simulink model "B5G_SIM_PDR_ASH_V0"  (R2021a)
settings: Solver=ode4  StartTime=0.0  StopTime=dm.duration  FixedStep=dm.dt  RelTol=1e-3
InitFcn:
  | %b5g_init_param_sdr_v1;
StopFcn:
  | %b5g_post_param_sdr_v1;
  | 
  | %if mdl.OpenAfterSim.sdi
  | %   Simulink.sdi.view;
  | %end
  | 
  | %if mdl.OpenAfterSim.Scope
  | %   open_system(strcat(gcs,'/RateRwTorque'));
  | %end
model workspace (MAT data in the model file):
  RWModelType = 0
values from neighbouring files (symbols this model uses):
  dm = set_dm(dm)    [INIT_B5G_SIM_PDR_ASH.m]
  mdl = set_model_control()    [INIT_B5G_SIM_PDR_ASH.m]    (also in init_b5g_sim_pdr.m = set_model_control('B5G_SIM_PDR_V1'))
  rads2rpm = 60/(2*pi)    (= 9.54929658551)    [INIT_B5G_SIM_PDR_ASH.m]    (also in init_b5g_sim_pdr.m)
undefined symbols (not defined in the file or in its folder): Eclipse, fsw, MagSc, PVeci, Qi2b, RateSc, SunSc
libraries: vrlib x2, aerolibtransform2 x1
(part 1 of 2)
settings Model: SimulationMode=accelerator  ParameterArgumentNames=RWModelType  OrderedModelArguments=off  Creator=Jack-AOCS  LastModifiedBy=jacky
settings SolverCC: AlgebraicLoopSolver=TrustRegion  MinimalZcImpactIntegration=on
settings DataIOCC: SaveFormat=Array
settings OptimizationCC: AccelVerboseBuild=on
settings DebuggingCC: ReadBeforeWriteMsg=DisableAll  WriteAfterWriteMsg=DisableAll  WriteAfterReadMsg=DisableAll  MultiTaskDSMMsg=none  SFMachineParentedDataDiag=warning  ArithmeticOperatorsInVariantConditions=warning
settings ModelReferenceCC: UpdateModelReferenceTargets=IfOutOfDate
settings SFSimCC: SFSimEcho=off  SimUseLocalCustomCode=off  CustomCodeUndefinedFunction=UseInterfaceOnly
settings RTWCC: RTWUseLocalCustomCode=off

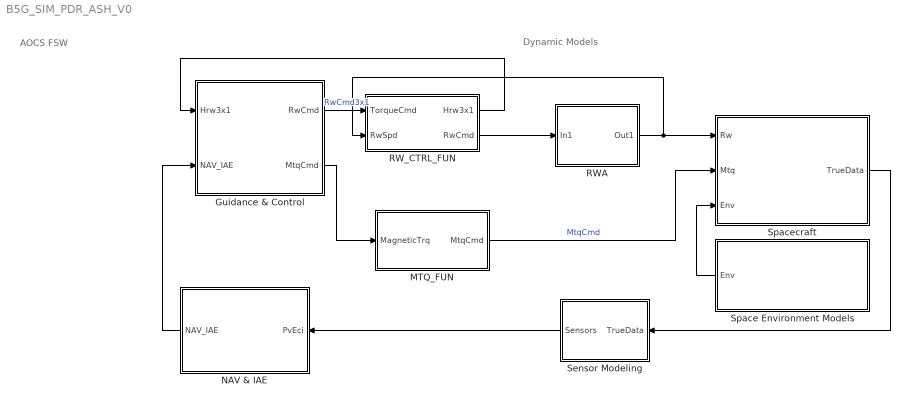
== system B5G_SIM_PDR_ASH_V0 ==
  note: AOCS FSW
  note: Dynamic Models
  Guidance & Control : Subsystem
  MTQ_FUN : Subsystem
  NAV & IAE : Subsystem
  RWA : Subsystem  Variant=on
  RW_CTRL_FUN : Subsystem
  Sensor Modeling : Subsystem
  Space Environment Models : Subsystem
  Spacecraft : Subsystem
  wires:
  Sensor Modeling/1(Sensors) -> NAV & IAE/1(PvEci)
  RWA/1(Out1) -> Spacecraft/1(Rw), RW_CTRL_FUN/2(RwSpd)
  Space Environment Models/1(Env) -> Spacecraft/3(Env)
  Spacecraft/1(TrueData) -> Sensor Modeling/1("TrueData ")
  RW_CTRL_FUN/2(RwCmd) -> RWA/1(In1)
  RW_CTRL_FUN/1(Hrw3x1) -> Guidance & Control/1(Hrw3x1)
  NAV & IAE/1(NAV_IAE) -> Guidance & Control/2(NAV_IAE)
  Guidance & Control/1(RwCmd) -> RW_CTRL_FUN/1(TorqueCmd)  "RwCmd3x1"
  Guidance & Control/2(MtqCmd) -> MTQ_FUN/1(MagneticTrq)
  MTQ_FUN/1(MtqCmd) -> Spacecraft/2(Mtq)  "MtqCmd"

== system B5G_SIM_PDR_ASH_V0/Guidance & Control ==
  Hrw3x1 : Inport
  NAV_IAE : Inport  Port=2
  ASH Mode : Subsystem
  RwCmd : Outport
  MtqCmd : Outport  Port=2
  wires:
  Hrw3x1/1 -> ASH Mode/1(Hrw3x1)
  NAV_IAE/1 -> ASH Mode/2(Sensors)
  ASH Mode/1(RwCmd) -> RwCmd/1  "RwTrq3"
  ASH Mode/2(MtqCmd) -> MtqCmd/1

== system B5G_SIM_PDR_ASH_V0/MTQ_FUN ==
  MagneticTrq : Inport
  Rate Transition : RateTransition  OutPortSampleTime=fsw.bdot_period
  Saturation : Saturate  UpperLimit=fsw.mtq.func.max_dipole  LowerLimit=-fsw.mtq.func.max_dipole
  MtqCmd : Outport
  wires:
  Rate Transition/1 -> Saturation/1
  Saturation/1 -> MtqCmd/1
  MagneticTrq/1 -> Rate Transition/1

== system B5G_SIM_PDR_ASH_V0/NAV & IAE ==
  PvEci : Inport
  Bus Creator : BusCreator  Inputs=2
  Bus Selector1 : BusSelector  OutputSignals=PVeci
  MATLAB Function : MATLAB Function  TreatAsAtomicUnit=on
  NAV_IAE : Outport
  wires:
  Bus Selector1/1 -> MATLAB Function/1(pv_eci)  "<PVeci>"
  PvEci/1 -> Bus Creator/2, Bus Selector1/1
  MATLAB Function/1(nav_out) -> Bus Creator/1
  Bus Creator/1 -> NAV_IAE/1

== system B5G_SIM_PDR_ASH_V0/RWA ==
  note: 1) Add Subsystem or Model blocks as valid variant choices.
      | 2) You cannot connect blocks at this level. At simulation, connectivity is automatically
      | determined, based on the active variant and port name matching.
  In1 : Inport
  Nonlinear : Subsystem  VariantControl=RWModel == 2
  Original : Subsystem  VariantControl=RWModel == 1
  Out1 : Outport

== system B5G_SIM_PDR_ASH_V0/RW_CTRL_FUN ==
  TorqueCmd : Inport
  RwSpd : Inport  Port=2
  Angular momentum Estimate : MATLAB Function  TreatAsAtomicUnit=on
  ComputeSaturate : MATLAB Function  TreatAsAtomicUnit=on
  D : Gain  Gain=fsw.rw.func.D  Multiplication=Matrix(K*u) (u vector)
  G : Gain  Gain=fsw.rw.func.G  Multiplication=Matrix(K*u) (u vector)
  RW Kernel Control : Subsystem
  Rate Transition : RateTransition  OutPortSampleTime=fsw.dt
  Sum2 : Sum  Inputs=|++
  Unit Delay : UnitDelay  SampleTime=-1  HasFrameUpgradeWarning=on
  Hrw3x1 : Outport
  RwCmd : Outport  Port=2
  wires:
  TorqueCmd/1 -> G/1
  RwSpd/1 -> Angular momentum Estimate/1(w_rpm)  "RwSpd"
  G/1 -> Sum2/1  "C_A"
  Sum2/1 -> ComputeSaturate/1(T)
  Angular momentum Estimate/1(h) -> D/1, RW Kernel Control/1(h_est)  "h_est"
  Unit Delay/1 -> Angular momentum Estimate/2(tc)
  RW Kernel Control/1(C_N) -> Sum2/2
  ComputeSaturate/1(Tc) -> Rate Transition/1, Unit Delay/1
  Rate Transition/1 -> RwCmd/1  "RwTrq4"
  D/1 -> Hrw3x1/1  "Hrw"

== system B5G_SIM_PDR_ASH_V0/Sensor Modeling ==
  "TrueData " : Inport
  Bus Creator : BusCreator  Inputs=5
  Bus Selector : BusSelector  OutputSignals=SunSc,Eclipse
  Bus Selector1 : BusSelector  OutputSignals=RateSc,Qi2b,MagSc,PVeci
  MATLAB Function : MATLAB Function  TreatAsAtomicUnit=on
  Sensors : Outport
  wires:
  "TrueData "/1 -> Bus Selector1/1, Bus Selector/1
  Bus Selector/1 -> MATLAB Function/1(SunSc)  "<SunSc>"
  Bus Selector/2 -> MATLAB Function/2(EclipFlag)  "<Eclipse>"
  MATLAB Function/1(SS_TM) -> Bus Creator/1
  Bus Selector1/1 -> Bus Creator/2  "<RateSc>"
  Bus Selector1/2 -> Bus Creator/3  "<Qi2b>"
  Bus Selector1/3 -> Bus Creator/4  "<MagSc>"
  Bus Selector1/4 -> Bus Creator/5  "<PVeci>"
  Bus Creator/1 -> Sensors/1

== system B5G_SIM_PDR_ASH_V0/Space Environment Models ==
  Bus Creator : BusCreator  Inputs=4
  ECI2ECF : MATLAB Function  TreatAsAtomicUnit=on
  Eclipse Condition : MATLAB Function  TreatAsAtomicUnit=on
  MagneticField : Subsystem
  Mux : Mux  Inputs=2
  "Orbit Propagator " : Subsystem
  Product : Product  Multiplication=Matrix(*)
  Sun Model : MATLAB Function  TreatAsAtomicUnit=on
  Timer : Subsystem
  Env : Outport  VectorParamsAs1DForOutWhenUnconnected=off
  wires:
  ECI2ECF/1(Rf2i) -> Product/1
  Product/1 -> Bus Creator/1  "Beci"
  "Orbit Propagator "/1(Peci) -> ECI2ECF/2(Peci), Mux/1
  "Orbit Propagator "/2(Veci) -> Mux/2
  Timer/1(JD) -> Sun Model/1(jD), ECI2ECF/1(jdut1)
  Mux/1 -> Eclipse Condition/2(PvEci), Bus Creator/4  "PVeci"
  Bus Creator/1 -> Env/1
  Sun Model/1(SunEci) -> Bus Creator/2, Eclipse Condition/1(SunEci)  "SunVeci"
  Eclipse Condition/1(EclipFlag) -> Bus Creator/3  "Eclipse"
  ECI2ECF/2(Pecf) -> MagneticField/1(In1)
  MagneticField/1(Out1) -> Product/2

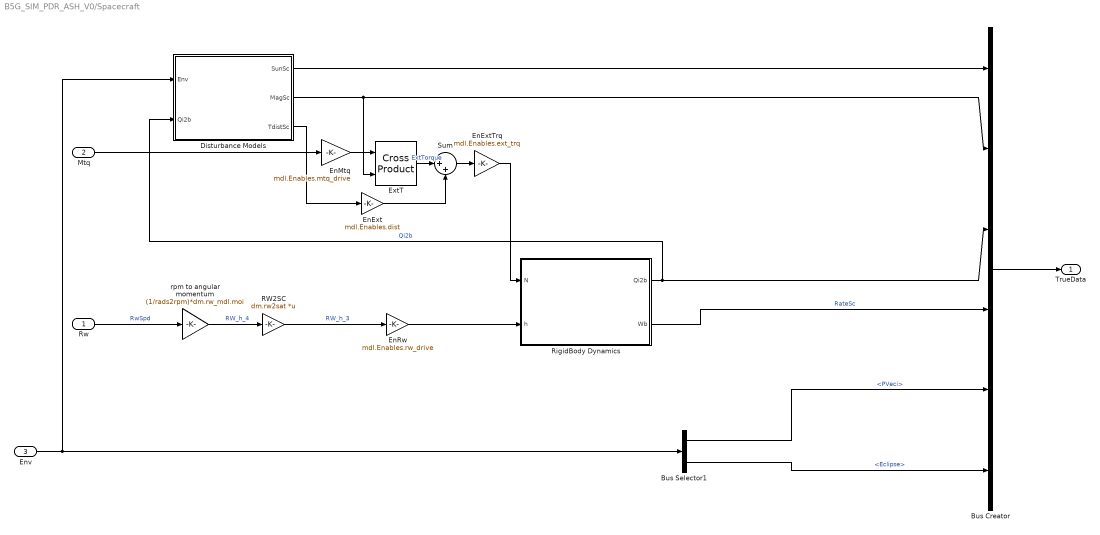
== system B5G_SIM_PDR_ASH_V0/Spacecraft ==
  Rw : Inport
  Mtq : Inport  Port=2
  Env : Inport  Port=3
  Bus Creator : BusCreator  Inputs=SunSc,MagSc,Qi2b,RateSc,PVeci,Eclipse
  Bus Selector1 : BusSelector  OutputSignals=PVeci,Eclipse
  Disturbance Models : Subsystem
  EnExt : Gain  Gain=mdl.Enables.dist
  EnExtTrq : Gain  Gain=mdl.Enables.ext_trq
  EnMtq : Gain  Gain=mdl.Enables.mtq_drive
  EnRw : Gain  Gain=mdl.Enables.rw_drive
  ExtT : vrlib/Utilities/Cross Product
  RW2SC : Gain  Gain=dm.rw2sat  Multiplication=Matrix(K*u)
  RigidBody Dynamics : Subsystem
  Sum : Sum  Inputs=|++
  rpm to angular momentum : Gain  Gain=(1/rads2rpm)*dm.rw_mdl.moi
  TrueData : Outport  VectorParamsAs1DForOutWhenUnconnected=off
  wires:
  ExtT/1 -> Sum/1  "ExtTorque"
  Sum/1 -> EnExtTrq/1
  RW2SC/1 -> EnRw/1  "RW_h_3"
  Disturbance Models/1(SunSc) -> Bus Creator/1
  Disturbance Models/3(TdistSc) -> EnExt/1
  Bus Selector1/2 -> Bus Creator/6  "<Eclipse>"
  Bus Selector1/1 -> Bus Creator/5  "<PVeci>"
  Env/1 -> Disturbance Models/1(Env), Bus Selector1/1
  RigidBody Dynamics/2(Wb) -> Bus Creator/4  "RateSc"
  rpm to angular momentum/1 -> RW2SC/1  "RW_h_4"
  Rw/1 -> rpm to angular momentum/1  "RwSpd"
  RigidBody Dynamics/1(Qi2b) -> Disturbance Models/2(Qi2b), Bus Creator/3  "Qi2b"
  Mtq/1 -> EnMtq/1
  Disturbance Models/2(MagSc) -> Bus Creator/2, ExtT/2
  EnExt/1 -> Sum/2
  EnMtq/1 -> ExtT/1
  Bus Creator/1 -> TrueData/1
  EnExtTrq/1 -> RigidBody Dynamics/1(N)
  EnRw/1 -> RigidBody Dynamics/2(h)

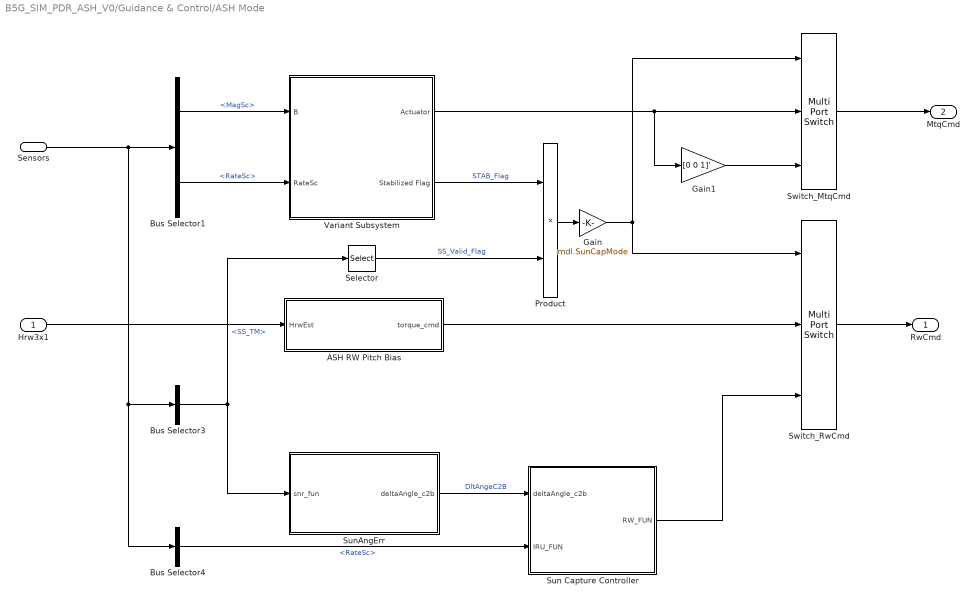
== system B5G_SIM_PDR_ASH_V0/Guidance & Control/ASH Mode ==
  Hrw3x1 : Inport
  Sensors : Inport  Port=2
  "ASH RW Pitch Bias " : Subsystem
  Bus Selector1 : BusSelector  OutputSignals=signal2.MagSc,signal2.RateSc
  Bus Selector3 : BusSelector  OutputSignals=signal2.SS_TM
  Bus Selector4 : BusSelector  OutputSignals=signal2.RateSc
  Gain : Gain  Gain=mdl.SunCapMode
  Gain1 : Gain  Gain=[0 0 1]'
  Product : Product
  Selector : Selector  InputPortWidth=4  IndexOptions=Index vector (dialog)  Indices=[4]  OutputSizes=1
  Sun Capture Controller : Subsystem
  SunAngErr : MATLAB Function  TreatAsAtomicUnit=on
  Switch_MtqCmd : MultiPortSwitch  DataPortOrder=Specify indices  DataPortIndices={0,1}  DiagnosticForDefault=None
  "Switch_RwCmd " : MultiPortSwitch  DataPortOrder=Specify indices  DataPortIndices={0,1}  DiagnosticForDefault=None
  Variant Subsystem : Subsystem  Variant=on
  RwCmd : Outport
  MtqCmd : Outport  Port=2
  wires:
  Sensors/1 -> Bus Selector4/1, Bus Selector3/1, Bus Selector1/1
  Bus Selector1/1 -> Variant Subsystem/1(B)  "<MagSc>"
  Hrw3x1/1 -> "ASH RW Pitch Bias "/1(HrwEst)
  Bus Selector3/1 -> SunAngErr/1(snr_fun), Selector/1  "<SS_TM>"
  "ASH RW Pitch Bias "/1(torque_cmd) -> "Switch_RwCmd "/2
  Variant Subsystem/1(Actuator) -> Switch_MtqCmd/2, Gain1/1
  "Switch_RwCmd "/1 -> RwCmd/1
  Selector/1 -> Product/2  "SS_Valid_Flag"
  Variant Subsystem/2(Stabilized Flag) -> Product/1  "STAB_Flag"
  Gain/1 -> "Switch_RwCmd "/1, Switch_MtqCmd/1
  Product/1 -> Gain/1
  Bus Selector1/2 -> Variant Subsystem/2(RateSc)  "<RateSc>"
  SunAngErr/1(deltaAngle_c2b) -> Sun Capture Controller/1(deltaAngle_c2b)  "DltAngeC2B"
  Bus Selector4/1 -> Sun Capture Controller/2(IRU_FUN)  "<RateSc>"
  Switch_MtqCmd/1 -> MtqCmd/1
  Gain1/1 -> Switch_MtqCmd/3
  Sun Capture Controller/1(RW_FUN) -> "Switch_RwCmd "/3

== system B5G_SIM_PDR_ASH_V0/RWA/Nonlinear ==
  In1 : Inport
  Demux : Demux
  Mux : Mux
  RW1 : Subsystem
  RW2 : Subsystem
  RW3 : Subsystem
  RW4 : Subsystem
  Out1 : Outport
  wires:
  RW1/1(Out1) -> Mux/1
  Demux/3 -> RW3/1(torque_cmd)
  RW2/1(Out1) -> Mux/2
  RW3/1(Out1) -> Mux/3
  Mux/1 -> Out1/1  "RW spd"
  Demux/4 -> RW4/1(torque_cmd)
  RW4/1(Out1) -> Mux/4
  Demux/1 -> RW1/1(torque_cmd)
  Demux/2 -> RW2/1(torque_cmd)
  In1/1 -> Demux/1

== system B5G_SIM_PDR_ASH_V0/RWA/Original ==
  In1 : Inport
  Demux : Demux
  Mux : Mux
  RW1 : Subsystem
  RW2 : Subsystem
  RW3 : Subsystem
  RW4 : Subsystem
  Out1 : Outport
  wires:
  RW4/1(Out1) -> Mux/4
  In1/1 -> Demux/1
  Mux/1 -> Out1/1  "RW spd"
  Demux/2 -> RW2/1(torque_cmd)
  Demux/4 -> RW4/1(torque_cmd)
  RW1/1(Out1) -> Mux/1
  Demux/1 -> RW1/1(torque_cmd)
  RW2/1(Out1) -> Mux/2
  RW3/1(Out1) -> Mux/3
  Demux/3 -> RW3/1(torque_cmd)

== system B5G_SIM_PDR_ASH_V0/RW_CTRL_FUN/RW Kernel Control ==
  h_est : Inport
  Kernel angular momentum(h_used) : Constant  Value=fsw.rw.func.KERNEL_ANG_MOM_REF
  Kernel direction : Gain  Gain=fsw.rw.func.K_KERNEL_DIRECTION
  Kernel momentum gain(h_used) : Gain  Gain=fsw.rw.func.KERNEL_ANG_MOM_GAIN
  Sum3 : Sum  Inputs=|+-
  kernal angular moementum : Gain  Gain=fsw.rw.func.E  Multiplication=Matrix(K*u) (u vector)
  C_N : Outport
  wires:
  Kernel angular momentum(h_used)/1 -> Kernel direction/1
  Kernel direction/1 -> Sum3/1  "hc"
  kernal angular moementum/1 -> Sum3/2
  Kernel momentum gain(h_used)/1 -> C_N/1  "C_N"
  Sum3/1 -> Kernel momentum gain(h_used)/1
  h_est/1 -> kernal angular moementum/1

== system B5G_SIM_PDR_ASH_V0/Space Environment Models/MagneticField ==
  In1 : Inport
  Variant Subsystem : Subsystem  Variant=on
  Out1 : Outport
  wires:
  In1/1 -> Variant Subsystem/1(Pecf)
  Variant Subsystem/1(BnT) -> Out1/1

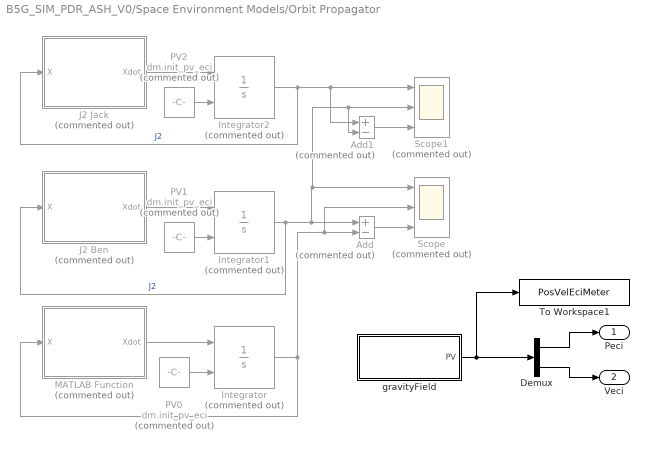
== system B5G_SIM_PDR_ASH_V0/Space Environment Models/Orbit Propagator  ==
  Add : Sum  Commented=on  Inputs=+-
  Add1 : Sum  Commented=on  Inputs=+-
  Demux : Demux  Outputs=2
  Integrator : Integrator  Commented=on  InitialConditionSource=external
  Integrator1 : Integrator  Commented=on  InitialConditionSource=external
  Integrator2 : Integrator  Commented=on  InitialConditionSource=external
  J2 Ben : MATLAB Function  Commented=on  TreatAsAtomicUnit=on
  J2 Jack : MATLAB Function  Commented=on  TreatAsAtomicUnit=on
  MATLAB Function : MATLAB Function  Commented=on  TreatAsAtomicUnit=on
  PV0 : Constant  Commented=on  Value=dm.init_pv_eci
  PV1 : Constant  Commented=on  Value=dm.init_pv_eci
  PV2 : Constant  Commented=on  Value=dm.init_pv_eci
  Scope : Scope  Commented=on  NumInputPorts=3
  Scope1 : Scope  Commented=on  NumInputPorts=3
  To Workspace1 : ToWorkspace  VariableName=PosVelEciMeter  SaveFormat=Timeseries  SampleTime=-1
  gravityField : Subsystem  Variant=on
  Peci : Outport  VectorParamsAs1DForOutWhenUnconnected=off
  Veci : Outport  Port=2  VectorParamsAs1DForOutWhenUnconnected=off
  wires:
  Demux/2 -> Veci/1
  MATLAB Function/1(Xdot) -> Integrator/1
  Integrator/1 -> Add/2, Scope/2, MATLAB Function/1(X)
  Demux/1 -> Peci/1
  PV0/1 -> Integrator/2
  PV1/1 -> Integrator1/2
  J2 Ben/1(Xdot) -> Integrator1/1
  Integrator1/1 -> J2 Ben/1(X), Add/1, Add1/2, Scope1/2, Scope/1  "J2"
  Add/1 -> Scope/3
  PV2/1 -> Integrator2/2
  J2 Jack/1(Xdot) -> Integrator2/1
  Integrator2/1 -> J2 Jack/1(X), Add1/1, Scope1/1  "J2"
  Add1/1 -> Scope1/3
  gravityField/1(PV) -> To Workspace1/1, Demux/1

== system B5G_SIM_PDR_ASH_V0/Space Environment Models/Timer ==
  Clock : Clock
  Constant : Constant  Value=dm.jd0
  Gain : Gain  Gain=1/86400
  Sum : Sum  Inputs=|++
  JD : Outport  VectorParamsAs1DForOutWhenUnconnected=off
  wires:
  Clock/1 -> Gain/1
  Gain/1 -> Sum/2
  Constant/1 -> Sum/1
  Sum/1 -> JD/1

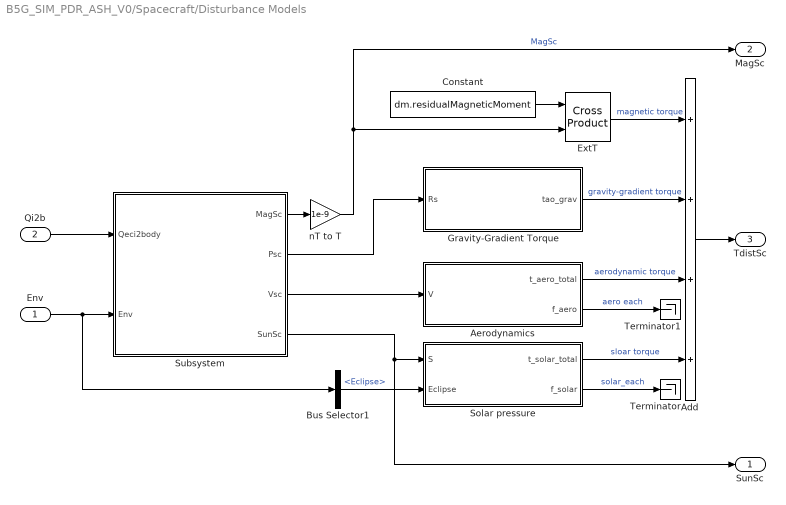
== system B5G_SIM_PDR_ASH_V0/Spacecraft/Disturbance Models ==
  Env : Inport
  Qi2b : Inport  Port=2
  Add : Sum  Inputs=4
  Aerodynamics : MATLAB Function  TreatAsAtomicUnit=on
  Bus Selector1 : BusSelector  OutputSignals=Eclipse
  Constant : Constant  Value=dm.residualMagneticMoment
  ExtT : vrlib/Utilities/Cross Product
  Gravity-Gradient Torque : MATLAB Function  TreatAsAtomicUnit=on
  Solar pressure : MATLAB Function  TreatAsAtomicUnit=on
  Subsystem : Subsystem
  Terminator : Terminator
  Terminator1 : Terminator
  nT to T : Gain  Gain=1e-9
  SunSc : Outport
  MagSc : Outport  Port=2
  TdistSc : Outport  Port=3
  wires:
  Gravity-Gradient Torque/1(tao_grav) -> Add/2  "gravity-gradient torque"
  Add/1 -> TdistSc/1
  Aerodynamics/2(f_aero) -> Terminator1/1  "aero each"
  Solar pressure/2(f_solar) -> Terminator/1  "solar_each"
  Env/1 -> Subsystem/2(Env), Bus Selector1/1
  Bus Selector1/1 -> Solar pressure/2(Eclipse)  "<Eclipse>"
  Qi2b/1 -> Subsystem/1(Qeci2body)
  Subsystem/2(Psc) -> Gravity-Gradient Torque/1(Rs)
  Subsystem/3(Vsc) -> Aerodynamics/1(V)
  Subsystem/4(SunSc) -> SunSc/1, Solar pressure/1(S)
  Aerodynamics/1(t_aero_total) -> Add/3  "aerodynamic torque"
  Solar pressure/1(t_solar_total) -> Add/4  "sloar torque"
  Constant/1 -> ExtT/1
  Subsystem/1(MagSc) -> nT to T/1
  ExtT/1 -> Add/1  "magnetic torque"
  nT to T/1 -> MagSc/1, ExtT/2  "MagSc"

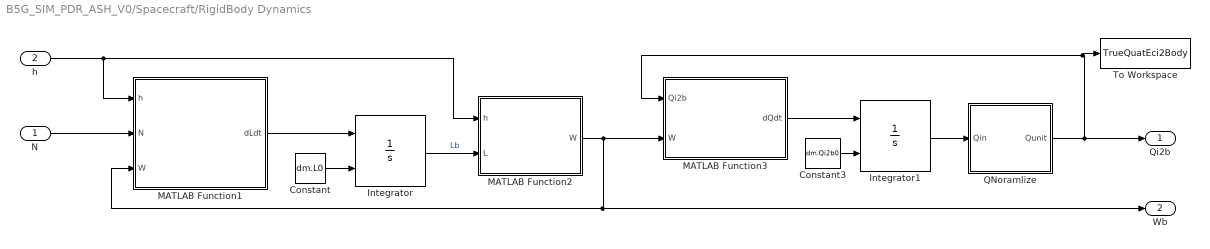
== system B5G_SIM_PDR_ASH_V0/Spacecraft/RigidBody Dynamics ==
  N : Inport
  h : Inport  Port=2
  Constant : Constant  Value=dm.L0
  Constant3 : Constant  Value=dm.Qi2b0
  Integrator : Integrator  InitialConditionSource=external
  Integrator1 : Integrator  InitialConditionSource=external
  MATLAB Function1 : MATLAB Function  TreatAsAtomicUnit=on
  MATLAB Function2 : MATLAB Function  TreatAsAtomicUnit=on
  MATLAB Function3 : MATLAB Function  TreatAsAtomicUnit=on
  QNoramlize : Subsystem
  To Workspace : ToWorkspace  VariableName=TrueQuatEci2Body  SaveFormat=Timeseries  SampleTime=-1
  Qi2b : Outport  VectorParamsAs1DForOutWhenUnconnected=off
  Wb : Outport  Port=2  VectorParamsAs1DForOutWhenUnconnected=off
  wires:
  Constant/1 -> Integrator/2
  N/1 -> MATLAB Function1/2(N)
  MATLAB Function1/1(dLdt) -> Integrator/1
  MATLAB Function3/1(dQdt) -> Integrator1/1
  Constant3/1 -> Integrator1/2
  MATLAB Function2/1(W) -> MATLAB Function3/2(W), Wb/1, MATLAB Function1/3(W)
  Integrator/1 -> MATLAB Function2/2(L)  "Lb"
  h/1 -> MATLAB Function2/1(h), MATLAB Function1/1(h)
  Integrator1/1 -> QNoramlize/1(Qin)
  QNoramlize/1(Qunit) -> Qi2b/1, To Workspace/1, MATLAB Function3/1(Qi2b)

== system B5G_SIM_PDR_ASH_V0/Guidance & Control/ASH Mode/ASH RW Pitch Bias  ==
  HrwEst : Inport
  Kernel momentum gain(H_used) : Gain  Gain=fsw.rw.func.KP
  Sum : Sum  Inputs=|+-
  zero_spd_cmd(H_used) : Constant  Value=fsw.rw.func.PITCH_BIAS
  torque_cmd : Outport
  wires:
  Sum/1 -> Kernel momentum gain(H_used)/1
  Kernel momentum gain(H_used)/1 -> torque_cmd/1  "torque_cmd"
  HrwEst/1 -> Sum/2  "Total angular moementum"
  zero_spd_cmd(H_used)/1 -> Sum/1

== system B5G_SIM_PDR_ASH_V0/Guidance & Control/ASH Mode/Sun Capture Controller ==
  note: SunCapture Controller Design
  deltaAngle_c2b : Inport
  IRU_FUN : Inport  Port=2
  KD : Gain  Gain=fsw.RLPD.kd
  KP : Gain  Gain=fsw.RLPD.kp
  Saturation : Saturate  UpperLimit=0.02  LowerLimit=-0.02
  Sum : Sum  Inputs=|++
  RW_FUN : Outport  VectorParamsAs1DForOutWhenUnconnected=off
  wires:
  Saturation/1 -> Sum/1  "CmdKp"
  KP/1 -> Saturation/1
  KD/1 -> RW_FUN/1  "CmdKd"
  Sum/1 -> KD/1
  deltaAngle_c2b/1 -> KP/1
  IRU_FUN/1 -> Sum/2

== system B5G_SIM_PDR_ASH_V0/Guidance & Control/ASH Mode/Variant Subsystem ==
  note: 1) Add Subsystem or Model blocks as valid variant choices.
      | 2) You cannot connect blocks at this level. At simulation, connectivity is automatically
      | determined, based on the active variant and port name matching.
  B : Inport
  RateSc : Inport  Port=2
  BdotTraditional : Subsystem  VariantControl=BdotControlType == 1
  BdotWithRate : Subsystem  VariantControl=BdotControlType == 2
  Actuator : Outport
  Stabilized Flag : Outport  Port=2

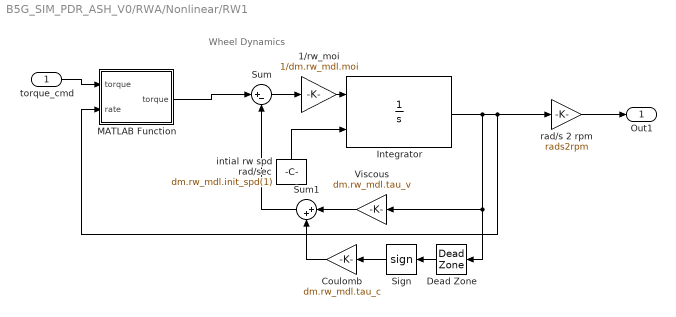
== system B5G_SIM_PDR_ASH_V0/RWA/Nonlinear/RW1 ==
  note: Wheel Dynamics
  torque_cmd : Inport
  1/rw_moi : Gain  Gain=1/dm.rw_mdl.moi
  Coulomb : Gain  Gain=dm.rw_mdl.tau_c
  Dead Zone : DeadZone  LowerValue=-dm.rw_mdl.dead_zone  UpperValue=dm.rw_mdl.dead_zone
  Integrator : Integrator  InitialConditionSource=external
  MATLAB Function : MATLAB Function  TreatAsAtomicUnit=on
  Sign : Signum
  Sum : Sum  Inputs=|+-
  Sum1 : Sum  Inputs=|++
  Viscous : Gain  Gain=dm.rw_mdl.tau_v
  intial rw spd rad/sec : Constant  Value=dm.rw_mdl.init_spd(1)
  rad/s 2 rpm : Gain  Gain=rads2rpm
  Out1 : Outport
  wires:
  Dead Zone/1 -> Sign/1
  Viscous/1 -> Sum1/1
  Integrator/1 -> MATLAB Function/2(rate), rad/s 2 rpm/1, Viscous/1, Dead Zone/1
  torque_cmd/1 -> MATLAB Function/1("torque ")
  Sum/1 -> 1/rw_moi/1
  intial rw spd rad/sec/1 -> Integrator/2
  Coulomb/1 -> Sum1/2
  Sign/1 -> Coulomb/1
  1/rw_moi/1 -> Integrator/1
  Sum1/1 -> Sum/2
  rad/s 2 rpm/1 -> Out1/1
  MATLAB Function/1(torque) -> Sum/1

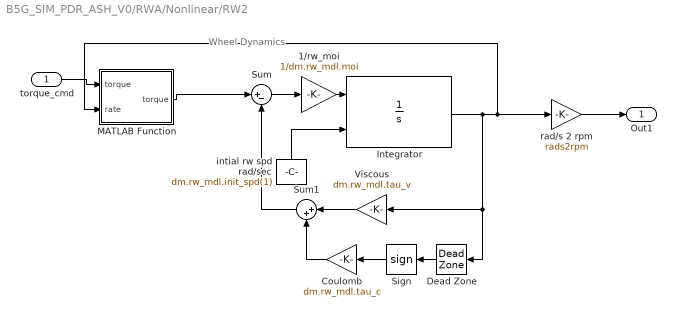
== system B5G_SIM_PDR_ASH_V0/RWA/Nonlinear/RW2 ==
  note: Wheel Dynamics
  torque_cmd : Inport
  1/rw_moi : Gain  Gain=1/dm.rw_mdl.moi
  Coulomb : Gain  Gain=dm.rw_mdl.tau_c
  Dead Zone : DeadZone  LowerValue=-dm.rw_mdl.dead_zone  UpperValue=dm.rw_mdl.dead_zone
  Integrator : Integrator  InitialConditionSource=external
  MATLAB Function : MATLAB Function  TreatAsAtomicUnit=on
  Sign : Signum
  Sum : Sum  Inputs=|+-
  Sum1 : Sum  Inputs=|++
  Viscous : Gain  Gain=dm.rw_mdl.tau_v
  intial rw spd rad/sec : Constant  Value=dm.rw_mdl.init_spd(1)
  rad/s 2 rpm : Gain  Gain=rads2rpm
  Out1 : Outport
  wires:
  Dead Zone/1 -> Sign/1
  Viscous/1 -> Sum1/1
  Integrator/1 -> MATLAB Function/2(rate), rad/s 2 rpm/1, Viscous/1, Dead Zone/1
  torque_cmd/1 -> MATLAB Function/1("torque ")
  Sum/1 -> 1/rw_moi/1
  intial rw spd rad/sec/1 -> Integrator/2
  Coulomb/1 -> Sum1/2
  Sign/1 -> Coulomb/1
  1/rw_moi/1 -> Integrator/1
  Sum1/1 -> Sum/2
  rad/s 2 rpm/1 -> Out1/1
  MATLAB Function/1(torque) -> Sum/1

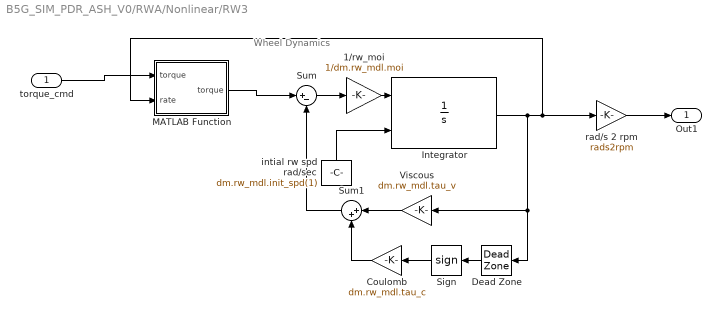
== system B5G_SIM_PDR_ASH_V0/RWA/Nonlinear/RW3 ==
  note: Wheel Dynamics
  torque_cmd : Inport
  1/rw_moi : Gain  Gain=1/dm.rw_mdl.moi
  Coulomb : Gain  Gain=dm.rw_mdl.tau_c
  Dead Zone : DeadZone  LowerValue=-dm.rw_mdl.dead_zone  UpperValue=dm.rw_mdl.dead_zone
  Integrator : Integrator  InitialConditionSource=external
  MATLAB Function : MATLAB Function  TreatAsAtomicUnit=on
  Sign : Signum
  Sum : Sum  Inputs=|+-
  Sum1 : Sum  Inputs=|++
  Viscous : Gain  Gain=dm.rw_mdl.tau_v
  intial rw spd rad/sec : Constant  Value=dm.rw_mdl.init_spd(1)
  rad/s 2 rpm : Gain  Gain=rads2rpm
  Out1 : Outport
  wires:
  Dead Zone/1 -> Sign/1
  Viscous/1 -> Sum1/1
  Integrator/1 -> MATLAB Function/2(rate), rad/s 2 rpm/1, Viscous/1, Dead Zone/1
  torque_cmd/1 -> MATLAB Function/1("torque ")
  Sum/1 -> 1/rw_moi/1
  intial rw spd rad/sec/1 -> Integrator/2
  Coulomb/1 -> Sum1/2
  Sign/1 -> Coulomb/1
  1/rw_moi/1 -> Integrator/1
  Sum1/1 -> Sum/2
  rad/s 2 rpm/1 -> Out1/1
  MATLAB Function/1(torque) -> Sum/1

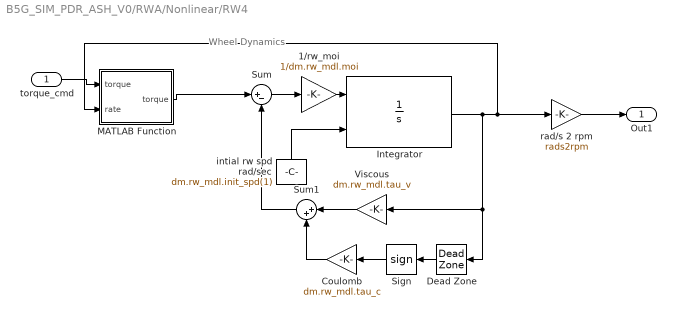
== system B5G_SIM_PDR_ASH_V0/RWA/Nonlinear/RW4 ==
  note: Wheel Dynamics
  torque_cmd : Inport
  1/rw_moi : Gain  Gain=1/dm.rw_mdl.moi
  Coulomb : Gain  Gain=dm.rw_mdl.tau_c
  Dead Zone : DeadZone  LowerValue=-dm.rw_mdl.dead_zone  UpperValue=dm.rw_mdl.dead_zone
  Integrator : Integrator  InitialConditionSource=external
  MATLAB Function : MATLAB Function  TreatAsAtomicUnit=on
  Sign : Signum
  Sum : Sum  Inputs=|+-
  Sum1 : Sum  Inputs=|++
  Viscous : Gain  Gain=dm.rw_mdl.tau_v
  intial rw spd rad/sec : Constant  Value=dm.rw_mdl.init_spd(1)
  rad/s 2 rpm : Gain  Gain=rads2rpm
  Out1 : Outport
  wires:
  Dead Zone/1 -> Sign/1
  Viscous/1 -> Sum1/1
  Integrator/1 -> MATLAB Function/2(rate), rad/s 2 rpm/1, Viscous/1, Dead Zone/1
  torque_cmd/1 -> MATLAB Function/1("torque ")
  Sum/1 -> 1/rw_moi/1
  intial rw spd rad/sec/1 -> Integrator/2
  Coulomb/1 -> Sum1/2
  Sign/1 -> Coulomb/1
  1/rw_moi/1 -> Integrator/1
  Sum1/1 -> Sum/2
  rad/s 2 rpm/1 -> Out1/1
  MATLAB Function/1(torque) -> Sum/1

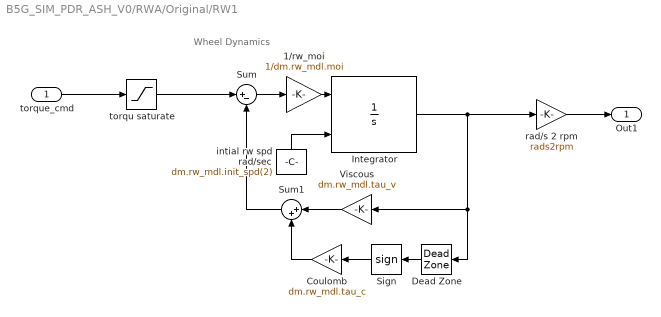
== system B5G_SIM_PDR_ASH_V0/RWA/Original/RW1 ==
  note: Wheel Dynamics
  torque_cmd : Inport
  1/rw_moi : Gain  Gain=1/dm.rw_mdl.moi
  Coulomb : Gain  Gain=dm.rw_mdl.tau_c
  Dead Zone : DeadZone  LowerValue=-dm.rw_mdl.dead_zone  UpperValue=dm.rw_mdl.dead_zone
  Integrator : Integrator  InitialConditionSource=external
  Sign : Signum
  Sum : Sum  Inputs=|+-
  Sum1 : Sum  Inputs=|++
  Viscous : Gain  Gain=dm.rw_mdl.tau_v
  intial rw spd rad/sec : Constant  Value=dm.rw_mdl.init_spd(2)
  rad/s 2 rpm : Gain  Gain=rads2rpm
  torqu saturate : Saturate  UpperLimit=dm.rw_mdl.maxTorque  LowerLimit=-dm.rw_mdl.maxTorque
  Out1 : Outport
  wires:
  rad/s 2 rpm/1 -> Out1/1
  Sum1/1 -> Sum/2
  torqu saturate/1 -> Sum/1
  1/rw_moi/1 -> Integrator/1
  Sign/1 -> Coulomb/1
  Coulomb/1 -> Sum1/2
  intial rw spd rad/sec/1 -> Integrator/2
  Sum/1 -> 1/rw_moi/1
  torque_cmd/1 -> torqu saturate/1
  Integrator/1 -> Dead Zone/1, Viscous/1, rad/s 2 rpm/1
  Viscous/1 -> Sum1/1
  Dead Zone/1 -> Sign/1

== system B5G_SIM_PDR_ASH_V0/RWA/Original/RW2 ==
  note: Wheel Dynamics
  torque_cmd : Inport
  1/rw_moi : Gain  Gain=1/dm.rw_mdl.moi
  Coulomb : Gain  Gain=dm.rw_mdl.tau_c
  Dead Zone : DeadZone  LowerValue=-dm.rw_mdl.dead_zone  UpperValue=dm.rw_mdl.dead_zone
  Integrator : Integrator  InitialConditionSource=external
  Sign : Signum
  Sum : Sum  Inputs=|+-
  Sum1 : Sum  Inputs=|++
  Viscous : Gain  Gain=dm.rw_mdl.tau_v
  intial rw spd rad/sec : Constant  Value=dm.rw_mdl.init_spd(2)
  rad/s 2 rpm : Gain  Gain=rads2rpm
  torqu saturate : Saturate  UpperLimit=dm.rw_mdl.maxTorque  LowerLimit=-dm.rw_mdl.maxTorque
  Out1 : Outport
  wires:
  Dead Zone/1 -> Sign/1
  Viscous/1 -> Sum1/1
  Integrator/1 -> rad/s 2 rpm/1, Viscous/1, Dead Zone/1
  torque_cmd/1 -> torqu saturate/1
  Sum/1 -> 1/rw_moi/1
  intial rw spd rad/sec/1 -> Integrator/2
  Coulomb/1 -> Sum1/2
  Sign/1 -> Coulomb/1
  1/rw_moi/1 -> Integrator/1
  torqu saturate/1 -> Sum/1
  Sum1/1 -> Sum/2
  rad/s 2 rpm/1 -> Out1/1

== system B5G_SIM_PDR_ASH_V0/RWA/Original/RW3 ==
  note: Wheel Dynamics
  torque_cmd : Inport
  1/rw_moi : Gain  Gain=1/dm.rw_mdl.moi
  Coulomb : Gain  Gain=dm.rw_mdl.tau_c
  Dead Zone : DeadZone  LowerValue=-dm.rw_mdl.dead_zone  UpperValue=dm.rw_mdl.dead_zone
  Integrator : Integrator  InitialConditionSource=external
  Sign : Signum
  Sum : Sum  Inputs=|+-
  Sum1 : Sum  Inputs=|++
  Viscous : Gain  Gain=dm.rw_mdl.tau_v
  intial rw spd rad/sec : Constant  Value=dm.rw_mdl.init_spd(3)
  rad/s 2 rpm : Gain  Gain=rads2rpm
  torqu saturate : Saturate  UpperLimit=dm.rw_mdl.maxTorque  LowerLimit=-dm.rw_mdl.maxTorque
  Out1 : Outport
  wires:
  Dead Zone/1 -> Sign/1
  Viscous/1 -> Sum1/1
  Integrator/1 -> rad/s 2 rpm/1, Viscous/1, Dead Zone/1
  torque_cmd/1 -> torqu saturate/1
  Sum/1 -> 1/rw_moi/1
  intial rw spd rad/sec/1 -> Integrator/2
  Coulomb/1 -> Sum1/2
  Sign/1 -> Coulomb/1
  1/rw_moi/1 -> Integrator/1
  torqu saturate/1 -> Sum/1
  Sum1/1 -> Sum/2
  rad/s 2 rpm/1 -> Out1/1

== system B5G_SIM_PDR_ASH_V0/RWA/Original/RW4 ==
  note: Wheel Dynamics
  torque_cmd : Inport
  1/rw_moi : Gain  Gain=1/dm.rw_mdl.moi
  Coulomb : Gain  Gain=dm.rw_mdl.tau_c
  Dead Zone : DeadZone  LowerValue=-dm.rw_mdl.dead_zone  UpperValue=dm.rw_mdl.dead_zone
  Integrator : Integrator  InitialConditionSource=external
  Sign : Signum
  Sum : Sum  Inputs=|+-
  Sum1 : Sum  Inputs=|++
  Viscous : Gain  Gain=dm.rw_mdl.tau_v
  intial rw spd rad/sec : Constant  Value=dm.rw_mdl.init_spd(4)
  rad/s 2 rpm : Gain  Gain=rads2rpm
  torqu saturate : Saturate  UpperLimit=dm.rw_mdl.maxTorque  LowerLimit=-dm.rw_mdl.maxTorque
  Out1 : Outport
  wires:
  Dead Zone/1 -> Sign/1
  Viscous/1 -> Sum1/1
  Integrator/1 -> rad/s 2 rpm/1, Viscous/1, Dead Zone/1
  torque_cmd/1 -> torqu saturate/1
  Sum/1 -> 1/rw_moi/1
  intial rw spd rad/sec/1 -> Integrator/2
  Coulomb/1 -> Sum1/2
  Sign/1 -> Coulomb/1
  1/rw_moi/1 -> Integrator/1
  torqu saturate/1 -> Sum/1
  Sum1/1 -> Sum/2
  rad/s 2 rpm/1 -> Out1/1

== system B5G_SIM_PDR_ASH_V0/Space Environment Models/MagneticField/Variant Subsystem ==
  note: 1) Add Subsystem or Model blocks as valid variant choices.
      | 2) You cannot connect blocks at this level. At simulation, connectivity is automatically
      | determined, based on the active variant and port name matching.
  Pecf : Inport
  IGRF2020 : Subsystem  VariantControl=M_IGRF
  MagneticDipoleModel : MATLAB Function  TreatAsAtomicUnit=on  VariantControl=M_DIPOLE
  BnT : Outport

== system B5G_SIM_PDR_ASH_V0/Space Environment Models/Orbit Propagator /gravityField ==
  note: 1) Add Subsystem or Model blocks as valid variant choices.
      | 2) You cannot connect blocks at this level. At simulation, connectivity is automatically
      | determined, based on the active variant and port name matching.
  J2 : Subsystem  VariantControl=G_J2
  TwoBodyRHS : Subsystem  VariantControl=G_TwoBody
  PV : Outport

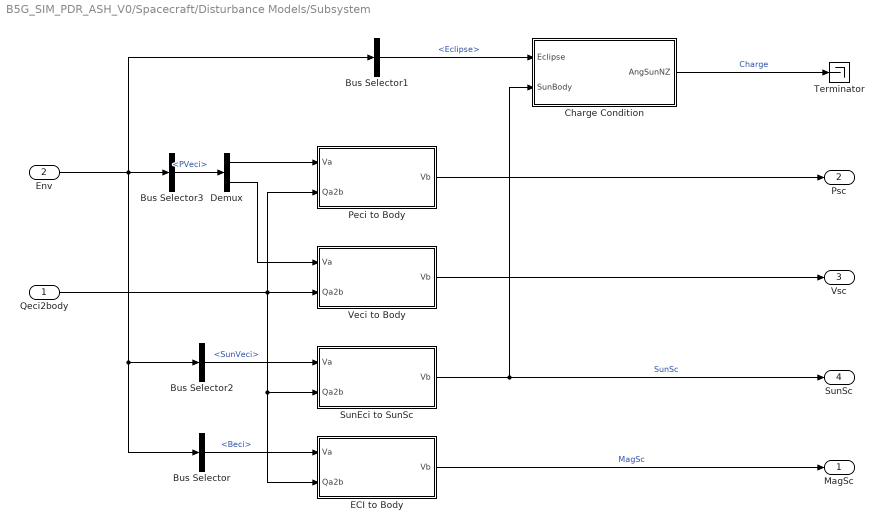
== system B5G_SIM_PDR_ASH_V0/Spacecraft/Disturbance Models/Subsystem ==
  Qeci2body : Inport
  Env : Inport  Port=2
  Bus Selector : BusSelector  OutputSignals=Beci
  Bus Selector1 : BusSelector  OutputSignals=Eclipse
  Bus Selector2 : BusSelector  OutputSignals=SunVeci
  Bus Selector3 : BusSelector  OutputSignals=PVeci
  Charge Condition : MATLAB Function  TreatAsAtomicUnit=on
  Demux : Demux  Outputs=2
  ECI to Body : MATLAB Function  TreatAsAtomicUnit=on
  Peci to Body : MATLAB Function  TreatAsAtomicUnit=on
  SunEci to SunSc : MATLAB Function  TreatAsAtomicUnit=on
  Terminator : Terminator
  Veci to Body : MATLAB Function  TreatAsAtomicUnit=on
  MagSc : Outport
  Psc : Outport  Port=2
  Vsc : Outport  Port=3
  SunSc : Outport  Port=4
  wires:
  Qeci2body/1 -> ECI to Body/2(Qa2b), SunEci to SunSc/2(Qa2b), Peci to Body/2(Qa2b), Veci to Body/2(Qa2b)
  Bus Selector/1 -> ECI to Body/1(Va)  "<Beci>"
  Peci to Body/1(Vb) -> Psc/1
  Bus Selector2/1 -> SunEci to SunSc/1(Va)  "<SunVeci>"
  ECI to Body/1(Vb) -> MagSc/1  "MagSc"
  Env/1 -> Bus Selector1/1, Bus Selector3/1, Bus Selector/1, Bus Selector2/1
  SunEci to SunSc/1(Vb) -> Charge Condition/2(SunBody), SunSc/1  "SunSc"
  Veci to Body/1(Vb) -> Vsc/1
  Bus Selector3/1 -> Demux/1  "<PVeci>"
  Demux/1 -> Peci to Body/1(Va)
  Demux/2 -> Veci to Body/1(Va)
  Bus Selector1/1 -> Charge Condition/1(Eclipse)  "<Eclipse>"
  Charge Condition/1(AngSunNZ) -> Terminator/1  "Charge"

== system B5G_SIM_PDR_ASH_V0/Spacecraft/RigidBody Dynamics/QNoramlize ==
  Qin : Inport
  Assertion : Assertion
  Divide : Product  Inputs=*/
  VectorNorm : Subsystem
  Qunit : Outport
  wires:
  Qin/1 -> VectorNorm/1(V), Divide/1
  Divide/1 -> Qunit/1
  VectorNorm/1(normV) -> Assertion/1, Divide/2

== system B5G_SIM_PDR_ASH_V0/Guidance & Control/ASH Mode/Variant Subsystem/BdotTraditional ==
  B : Inport
  RateSc : Inport  Port=2
  Bdot Control : MATLAB Function  TreatAsAtomicUnit=on
  MATLAB Function : MATLAB Function  TreatAsAtomicUnit=on
  Terminator : Terminator
  Terminator1 : Terminator
  Unit Delay : UnitDelay  SampleTime=-1  HasFrameUpgradeWarning=on
  Unit Delay1 : UnitDelay  InitialCondition=fsw.mtq.func.Count_stab  SampleTime=-1  HasFrameUpgradeWarning=on
  Unit Delay2 : UnitDelay  InitialCondition=fsw.mtq.func.Stabilized  SampleTime=-1  HasFrameUpgradeWarning=on
  Actuator : Outport  VectorParamsAs1DForOutWhenUnconnected=off
  Stabilized Flag : Outport  Port=2  VectorParamsAs1DForOutWhenUnconnected=off
  wires:
  Unit Delay/1 -> Bdot Control/2(B_1)
  B/1 -> Bdot Control/1(B), Unit Delay/1  "Bbody_tesla"
  MATLAB Function/2(Count_stab) -> Unit Delay1/1  "Count_stab"
  MATLAB Function/3(Stabilized) -> Stabilized Flag/1, Unit Delay2/1  "Stabilized"
  MATLAB Function/1(bdot_norm) -> Terminator/1  "bdot_norm"
  Unit Delay1/1 -> MATLAB Function/2("Count_stab ")
  Unit Delay2/1 -> MATLAB Function/3("Stabilized ")
  RateSc/1 -> Terminator1/1
  Bdot Control/1(Mc) -> Actuator/1  "M"
  Bdot Control/2(bdot) -> MATLAB Function/1(bdot)

== system B5G_SIM_PDR_ASH_V0/Guidance & Control/ASH Mode/Variant Subsystem/BdotWithRate ==
  B : Inport
  RateSc : Inport  Port=2
  BdotWithRate : MATLAB Function  TreatAsAtomicUnit=on
  MATLAB Function : MATLAB Function  TreatAsAtomicUnit=on
  Terminator : Terminator
  Unit Delay1 : UnitDelay  InitialCondition=fsw.mtq.func.Count_stab  SampleTime=-1  HasFrameUpgradeWarning=on
  Unit Delay2 : UnitDelay  InitialCondition=fsw.mtq.func.Stabilized  SampleTime=-1  HasFrameUpgradeWarning=on
  Actuator : Outport  VectorParamsAs1DForOutWhenUnconnected=off
  Stabilized Flag : Outport  Port=2  VectorParamsAs1DForOutWhenUnconnected=off
  wires:
  RateSc/1 -> BdotWithRate/2(RateSc)
  Unit Delay2/1 -> MATLAB Function/3("Stabilized ")
  Unit Delay1/1 -> MATLAB Function/2("Count_stab ")
  MATLAB Function/1(bdot_norm) -> Terminator/1  "bdot_norm"
  MATLAB Function/3(Stabilized) -> Unit Delay2/1, Stabilized Flag/1  "Stabilized"
  MATLAB Function/2(Count_stab) -> Unit Delay1/1  "Count_stab"
  B/1 -> BdotWithRate/1(Bb)  "Bbody_tesla"
  BdotWithRate/1(Mc) -> Actuator/1  "M"
  BdotWithRate/2(bdot) -> MATLAB Function/1(bdot)

== system B5G_SIM_PDR_ASH_V0/Space Environment Models/MagneticField/Variant Subsystem/IGRF2020 ==
  Pecf : Inport
  Constant : Constant  Value=dm.epoch.utc(1)
  Demux : Demux  Outputs=2
  Direction Cosine Matrix ECEF to NED : aerolibtransform2/Direction Cosine Matrix ECEF to NED
      settings: SourceProductBaseCode=AE
  ECEF Position to LLA : ECEF2LLA  R=6378137
  IGRF_ned2ecef : MATLAB Function  TreatAsAtomicUnit=on
  International Geomagnetic Reference Field : IGRF  month=January  day=1  year=2020
      settings: AttributesFormatString=%<generation>
  Mux1 : Mux  Inputs=9
  Scope : Scope
  Terminator : Terminator
  To Workspace : ToWorkspace  Commented=on  VariableName=MagEcef7Days  SaveFormat=Timeseries  SampleTime=-1
  BnT : Outport  VectorParamsAs1DForOutWhenUnconnected=off
  wires:
  International Geomagnetic Reference Field/7 -> Mux1/6
  International Geomagnetic Reference Field/4 -> Mux1/3
  International Geomagnetic Reference Field/3 -> Mux1/2
  International Geomagnetic Reference Field/6 -> Mux1/5
  International Geomagnetic Reference Field/5 -> Mux1/4
  International Geomagnetic Reference Field/9 -> Mux1/8
  International Geomagnetic Reference Field/8 -> Mux1/7
  International Geomagnetic Reference Field/10 -> Mux1/9
  Pecf/1 -> ECEF Position to LLA/1
  Mux1/1 -> Terminator/1
  International Geomagnetic Reference Field/2 -> Mux1/1
  ECEF Position to LLA/1 -> Demux/1, Direction Cosine Matrix ECEF to NED/1
  ECEF Position to LLA/2 -> International Geomagnetic Reference Field/1
  Constant/1 -> International Geomagnetic Reference Field/4
  Demux/1 -> International Geomagnetic Reference Field/2
  Demux/2 -> International Geomagnetic Reference Field/3
  Direction Cosine Matrix ECEF to NED/1 -> IGRF_ned2ecef/1(DCM)
  IGRF_ned2ecef/1(Vecef) -> To Workspace/1, BnT/1
  International Geomagnetic Reference Field/1 -> IGRF_ned2ecef/2(Vned), Scope/1

== system B5G_SIM_PDR_ASH_V0/Space Environment Models/Orbit Propagator /gravityField/J2 ==
  Integrator2 : Integrator  InitialConditionSource=external
  J2 Jack : MATLAB Function  TreatAsAtomicUnit=on
  PV2 : Constant  Value=dm.init_pv_eci
  PV : Outport
  wires:
  Integrator2/1 -> PV/1, J2 Jack/1(X)  "J2"
  J2 Jack/1(Xdot) -> Integrator2/1
  PV2/1 -> Integrator2/2

== system B5G_SIM_PDR_ASH_V0/Space Environment Models/Orbit Propagator /gravityField/TwoBodyRHS ==
  Integrator : Integrator  InitialConditionSource=external
  MATLAB Function : MATLAB Function  TreatAsAtomicUnit=on
  PV0 : Constant  Value=dm.init_pv_eci
  PV : Outport
  wires:
  Integrator/1 -> PV/1, MATLAB Function/1(X)  "TwoBody"
  MATLAB Function/1(Xdot) -> Integrator/1
  PV0/1 -> Integrator/2

== system B5G_SIM_PDR_ASH_V0/Spacecraft/RigidBody Dynamics/QNoramlize/VectorNorm ==
  V : Inport
  Dot Product1 : DotProduct  InputSameDT=on  OutDataTypeStr=Inherit: Inherit via internal rule
  Square Root1 : Sqrt  SaturateOnIntegerOverflow=on
  normV : Outport
  wires:
  Dot Product1/1 -> Square Root1/1
  V/1 -> Dot Product1/2, Dot Product1/1
  Square Root1/1 -> normV/1

== matlab function B5G_SIM_PDR_ASH_V0/Sensor Modeling/MATLAB Function ==
  data: SunSc input; SS_TM output; EclipFlag input; dm parameter
function SS_TM  = SunSensor(SunSc, EclipFlag, dm)
coder.extrinsic('randn');%%https://www.mathworks.com/matlabcentral/answers/385475-why-do-calls-to-randn-in-separate-matlab-function-blocks-return-the-same-sequence-of-random-number

if EclipFlag~=1
    %% Sun Sensor Modeling by Rodrigues Rotation Formula
    acc_1_sigma = (0.3/3)*pi/180;%0.3 deg in 3-sigma from Solar MEMS type xx
    n1 = zeros(3, 1);% Eigen Axis
    theta1 = zeros(1);
    
    n1 = randn(3, 1);
    n1 = n1/norm(n1);
    theta1 = acc_1_sigma * randn(1, 1);
    
    R1 = EigRotMatrix(n1, theta1);
%     SunSc_noise = R1*SunSc; %noisy sun vector
    SunSc_noise = SunSc; %Turn off SS noise model
    
    
    ang_ss1 = acos(dot(SunSc_noise, dm.ss1_mdl.los));
    ang_ss2 = acos(dot(SunSc_noise, dm.ss2_mdl.los));
    
    if ang_ss1 < dm.ss_mdl.fov || ang_ss2 < dm.ss_mdl.fov
        Valid = 1;
    else
        Valid = 0;
    end
else
    Valid = 0;
    SunSc_noise = zeros(3, 1);
end

SS_TM =[SunSc_noise; Valid];

end

%% Eigen Axis Rotation by Rodrigues Rotation Formula
function R = EigRotMatrix(n, theta)
nx = [	0       -n(3)	n(2);...
    n(3)	0       -n(1);...
    -n(2)	n(1)    0	];
R  = cos(theta)*eye(3)+(1-cos(theta))*(n*n')-sin(theta)*nx;
end

== matlab function B5G_SIM_PDR_ASH_V0/Space Environment Models/Eclipse Condition ==
  data: SunEci input; EclipFlag output; PvEci input
function EclipFlag  = Eclipse(SunEci, PvEci)
Dp = -PvEci(1:3)*1e-3;  % earth vector in Km
Rp = 6378.137;          % earth radius in km
Rs = 6.9599e5;          % solar photosphere radius in km
S  = 1.49597870e8;      % astronomical unit in km
C  = 1.385e6;           % size of earth shadow cone
Ds = (S.*SunEci + Dp);  % vector from S/C to the Sun

DsNorm = norm(Ds);
DpNorm = norm(Dp);
rho_s  = asind(Rs/DsNorm);
rho_p  = asind(Rp/DpNorm);
theta  = acosd(dot(Ds, Dp) / (DsNorm * DpNorm));
if ( theta < (rho_p - rho_s) && DsNorm > S && (S + C) > DsNorm)
    EclipFlag = 1;
else
	EclipFlag = 0;
end

== matlab function B5G_SIM_PDR_ASH_V0/Space Environment Models/Sun Model ==
  data: jD input; SunEci output
function SunEci = SunModel(jD)
T = JDCentury(jD);
lamda_mean     = rem(280.460+36000.771*T,360);
mean_anomaly   = rem(357.5291092+35999.05034*T,360);
lamda_ecliptic = lamda_mean+ 1.914666471*sind(mean_anomaly)...
                 + 0.019994643*sind(2*mean_anomaly);
% Obliquity of ecliptic
epsilon = 23.439291 -0.0130042*T;
SunEci  = [cosd(lamda_ecliptic);...
           cosd(epsilon)*sind(lamda_ecliptic);...
           sind(epsilon)*sind(lamda_ecliptic)];

== matlab function B5G_SIM_PDR_ASH_V0/NAV & IAE/MATLAB Function ==
  data: pv_eci input; nav_out output
function nav_out  = Navgation(pv_eci)

omega_orbit = OrbitPusaltion(pv_eci);
Qi2l        = PVi2Qi2l(pv_eci);
nav_out     = [omega_orbit; Qi2l];

== matlab function B5G_SIM_PDR_ASH_V0/Spacecraft/Disturbance Models/Subsystem/Peci to Body ==
  data: Va input; Qa2b input; Vb output
function Vb = EciToBody(Va,Qa2b)
Qb2a = QInv(Qa2b);
qout = QMul(QMul(Qb2a, [0;Va]), Qa2b);
Vb   = [qout(2) qout(3) qout(4)]';

== matlab function B5G_SIM_PDR_ASH_V0/Spacecraft/Disturbance Models/Subsystem/Veci to Body ==
  data: Va input; Qa2b input; Vb output
function Vb = EciToBody(Va,Qa2b)
Qb2a = QInv(Qa2b);
qout = QMul(QMul(Qb2a, [0;Va]), Qa2b);
Vb   = [qout(2) qout(3) qout(4)]';

== matlab function B5G_SIM_PDR_ASH_V0/Spacecraft/RigidBody Dynamics/MATLAB Function1 ==
  data: h input; dLdt output size=3; N input; W input; dm parameter
%% Euler Equation
function dLdt = EulerEquation(h,N,W,dm)
L = dm.Ib*W + h;
dLdt = N-cross((dm.Ib\(L-h)),L);

== matlab function B5G_SIM_PDR_ASH_V0/Spacecraft/RigidBody Dynamics/MATLAB Function2 ==
  data: h input; W output; L input; dm parameter
%% total angular momentum of the spacecraft
function W = InvTotAngMom(h,L,dm)
W =dm.Ib\(L-h);

== matlab function B5G_SIM_PDR_ASH_V0/Space Environment Models/ECI2ECF ==
  data: Rf2i output; jdut1 input; Pecf output; Peci input
%% ECI to ECEF Transformation
function [Rf2i, Pecf]  = ECI2ECF(jdut1, Peci)
Ri2f  = R3(JD2GMST(jdut1));
Pecf  = Ri2f*Peci; %in m
Rf2i  = Ri2f';

== matlab function B5G_SIM_PDR_ASH_V0/Spacecraft/RigidBody Dynamics/MATLAB Function3 ==
  data: Qi2b input; dQdt output size=4; W input
%% Quaternion Kinematic Equation
function dQdt = QuatKinematic(Qi2b,W)

dQdt = 0.5 * (QMul(Qi2b,[0;W]));

== matlab function B5G_SIM_PDR_ASH_V0/Space Environment Models/MagneticField/Variant Subsystem/IGRF2020/IGRF_ned2ecef ==
  data: DCM input; Vecef output; Vned input
function Vecef = fcn(DCM,Vned)

Vecef = DCM'*Vned;

== matlab function B5G_SIM_PDR_ASH_V0/Guidance & Control/ASH Mode/Variant Subsystem/BdotTraditional/Bdot Control ==
  settings: updateMethod=DISCRETE
  data: B input; Mc output; B_1 input; fsw parameter; bdot output
%% Bdot Control Rev
function [Mc,bdot] = Bdot(B, B_1, fsw)

mag   = norm(B);

if mag~=0 && norm(B_1)~=0 %this is a poka-yoke
    b   =  B/norm(B);
    b_1 =  B_1/norm(B_1);
    bdot = (b-b_1)/fsw.dt;
    sdot = (bdot-dot(b,bdot).*b)/norm(B);
    Mc = -fsw.bdot_gain.*sdot;
else
    Mc = zeros(3,1);
    bdot =zeros(3,1);
%     return;
end

== matlab function B5G_SIM_PDR_ASH_V0/Guidance & Control/ASH Mode/Variant Subsystem/BdotTraditional/MATLAB Function ==
  data: bdot_norm output; bdot input; Count_stab input; Stabilized input; Count_stab output; Stabilized output; fsw parameter
function [bdot_norm, Count_stab, Stabilized] = fcn(bdot,Count_stab, Stabilized, fsw)
    bdot_norm = norm(bdot);
    if Stabilized == 0
        if bdot_norm < fsw.ash_mgr.epsilon
            Count_stab = Count_stab + 1;
        else
            Count_stab = 0;
        end
        if Count_stab > fsw.ash_mgr.Tstab
            Stabilized = 1;
        end
    end

== matlab function B5G_SIM_PDR_ASH_V0/Spacecraft/Disturbance Models/Subsystem/Charge Condition ==
  data: Eclipse input; SunBody input; AngSunNZ output
 function AngSunNZ  = ChargeStatus(Eclipse, SunBody)
NZBody = [0 0 -1];
ang = acosd(dot(SunBody, NZBody));

if ( Eclipse ~= 1 && ang < 90 && ang > 0)
    AngSunNZ = ang;
else
    AngSunNZ = 0;
end

end

== matlab function B5G_SIM_PDR_ASH_V0/Guidance & Control/ASH Mode/SunAngErr ==
  data: deltaAngle_c2b output; snr_fun input
function deltaAngle_c2b = RPLD_CTRL_PROC(snr_fun)

if ~snr_fun(4) 
    deltaAngle_c2b = [0;0;0];
    return;
end

vec_sun_b = snr_fun(1:3);
mag = norm(vec_sun_b);
if mag~=0
    vec_sun_b = vec_sun_b/mag;
end

%% DCM to Euler Angle Method
zb = (-1)*vec_sun_b';
yb = [0 vec_sun_b(3) -vec_sun_b(2)];
xb = cross(yb,zb);
R_B2C = [xb;yb;zb];

theta_c2b = -asin(R_B2C(3, 1));
phi_c2b = atan(R_B2C(3, 2) / R_B2C(3, 3));
% psi_c2b = atan2(R_B2C(2, 1), R_B2C(1, 1)); //3.14
psi_c2b = atan(R_B2C(2, 1) / R_B2C(1, 1));

%% deltaAngle_c2b = deltaAngle_b/c = -deltaAngle_c/b = -deltaAngle_b2c
deltaAngle_c2b = [phi_c2b; theta_c2b; psi_c2b];

== matlab function B5G_SIM_PDR_ASH_V0/Guidance & Control/ASH Mode/Variant Subsystem/BdotWithRate/MATLAB Function ==
  data: bdot_norm output; bdot input; Count_stab input; Stabilized input; Count_stab output; Stabilized output; fsw parameter
function [bdot_norm, Count_stab, Stabilized] = fcn(bdot,Count_stab, Stabilized, fsw)
    bdot_norm = norm(bdot);
    if Stabilized == 0
        if bdot_norm < fsw.ash_mgr.epsilon
            Count_stab = Count_stab + 1;
        else
            Count_stab = 0;
        end
        if Count_stab > fsw.ash_mgr.Tstab
            Stabilized = 1;
        end
    end

== matlab function B5G_SIM_PDR_ASH_V0/Guidance & Control/ASH Mode/Variant Subsystem/BdotWithRate/BdotWithRate ==
  settings: updateMethod=DISCRETE
  data: Bb input; Mc output size=3; fsw parameter; bdot output size=3; RateSc input
%% BdotControl
function [Mc,bdot] = Bdot2(Bb, fsw, RateSc)

Bdot= -cross(RateSc,Bb);
nBdot= norm(Bdot);

%% divided-by-zero check
if abs(nBdot-eps)> 1e-10
    bdot= Bdot/norm(Bb); %% Correction: Fix Tutorial Typo
else
    bdot= zeros(3,1);
end

Mc = -fsw.wXbdot_gain .* bdot;

end

== matlab function B5G_SIM_PDR_ASH_V0/Space Environment Models/Orbit Propagator /J2 Ben ==
  data: X input; Xdot output; dm parameter
function Xdot = J2(X, dm)

r = X(1:3);
v = X(4:6);
J2 = 0.484165143790815D-03*(5)^0.5;
GMe = 3.986004418e14;                % m^3*s^-2
Re = 6378137;                        % earth radius, m
k_1_2 = -GMe/norm(r)^3 * (1+ 1.5 *J2* (Re/norm(r))^2 * (1 - 5* (r(3)/norm(r))^2) );
k_3 = -GMe/norm(r)^3 * (1+ 1.5 *J2* (Re/norm(r))^2 * (3 - 5* (r(3)/norm(r))^2) );
a = [k_1_2*r(1); k_1_2*r(2); k_3*r(3)];
Xdot=[v; a];

% Re   = 6378137.00;%m
% mu_e = 3.986004418e14;%3.986004418e14;
% 
% p = X(1:3);
% v = X(4:6);
% R = norm(p);
% 
% 
% J2 = 0.001082626173852;%0.001082626173852;% C20_bar = -0.484165143790815D-03 from EGM2008
% %0.001082626683553151; STK
%      
% ReOverR_2 = (Re/R)^2;
% sinphi_2   = (p(3)/R)^2;
% muOverR_3 = mu_e/R^3;
% vdot=[-muOverR_3*(1+1.5*J2*ReOverR_2*(1-5*sinphi_2));...
%       -muOverR_3*(1+1.5*J2*ReOverR_2*(1-5*sinphi_2));...
%       -muOverR_3*(1+1.5*J2*ReOverR_2*(3-5*sinphi_2))].*p;
%      
% Xdot=[v; vdot];

== matlab function B5G_SIM_PDR_ASH_V0/Space Environment Models/Orbit Propagator /MATLAB Function ==
  data: X input; Xdot output; dm parameter
function Xdot = TwoBodyRHS(X, dm)

r = X(1:3);
v = X(4:6);
Xdot=[v; -(dm.mu_e*r/norm(r)^3)];

== matlab function B5G_SIM_PDR_ASH_V0/Space Environment Models/Orbit Propagator /J2 Jack ==
  data: X input; Xdot output; dm parameter
function Xdot = J2(X, dm)

Re   = 6378137.00;%m
mu_e = 3.986004418e14;%3.986004418e14;

p = X(1:3);
v = X(4:6);
R = norm(p);


J2 = 0.001082626173852;%0.001082626173852;% C20_bar = -0.484165143790815D-03 from EGM2008
%0.001082626683553151; STK
     
ReOverR_2 = (Re/R)^2;
sinphi_2   = (p(3)/R)^2;
muOverR_3 = mu_e/R^3;
vdot=[-muOverR_3*(1+1.5*J2*ReOverR_2*(1-5*sinphi_2));...
      -muOverR_3*(1+1.5*J2*ReOverR_2*(1-5*sinphi_2));...
      -muOverR_3*(1+1.5*J2*ReOverR_2*(3-5*sinphi_2))].*p;
     
Xdot=[v; vdot];

== matlab function B5G_SIM_PDR_ASH_V0/RWA/Nonlinear/RW1/MATLAB Function ==
  data: torque input; torque output; rate input; dm parameter
function torque = torqueBox(torque,rate, dm)

momentum = dm.rw_mdl.moi * rate;
maxAngMom = dm.rw_mdl.maxAngMom;
AvlAngMom = dm.rw_mdl.avlAngMom;
maxTorque = dm.rw_mdl.maxTorque;

if momentum >= AvlAngMom && momentum <= maxAngMom
    torque = 1 + (-maxTorque) * (momentum);
elseif momentum <= -AvlAngMom && momentum >= (-maxAngMom)
    torque = -1 + (-maxTorque) * (momentum);
end

== matlab function B5G_SIM_PDR_ASH_V0/RWA/Nonlinear/RW2/MATLAB Function ==
  data: torque input; torque output; rate input; dm parameter
function torque = torqueBox(torque,rate, dm)

momentum = dm.rw_mdl.moi * rate;
maxAngMom = dm.rw_mdl.maxAngMom;
AvlAngMom = dm.rw_mdl.avlAngMom;
maxTorque = dm.rw_mdl.maxTorque;

if momentum >= AvlAngMom && momentum <= maxAngMom
    torque = 1 + (-maxTorque) * (momentum);
elseif momentum <= -AvlAngMom && momentum >= (-maxAngMom)
    torque = -1 + (-maxTorque) * (momentum);
end

== matlab function B5G_SIM_PDR_ASH_V0/Space Environment Models/Orbit Propagator /gravityField/TwoBodyRHS/MATLAB Function ==
  data: X input; Xdot output; dm parameter
function Xdot = TwoBodyRHS(X, dm)

r = X(1:3);
v = X(4:6);
Xdot=[v; -(dm.mu_e*r/norm(r)^3)];

== matlab function B5G_SIM_PDR_ASH_V0/Space Environment Models/Orbit Propagator /gravityField/J2/J2 Jack ==
  data: X input; Xdot output; dm parameter
function Xdot = J2(X, dm)

Re   = 6378137.00;%m
mu_e = 3.986004418e14;%3.986004418e14;

p = X(1:3);
v = X(4:6);
R = norm(p);


J2 = 0.001082626173852;%0.001082626173852;% C20_bar = -0.484165143790815D-03 from EGM2008
%0.001082626683553151; STK
     
ReOverR_2 = (Re/R)^2;
sinphi_2   = (p(3)/R)^2;
muOverR_3 = mu_e/R^3;
vdot=[-muOverR_3*(1+1.5*J2*ReOverR_2*(1-5*sinphi_2));...
      -muOverR_3*(1+1.5*J2*ReOverR_2*(1-5*sinphi_2));...
      -muOverR_3*(1+1.5*J2*ReOverR_2*(3-5*sinphi_2))].*p;
     
Xdot=[v; vdot];

== matlab function B5G_SIM_PDR_ASH_V0/RWA/Nonlinear/RW3/MATLAB Function ==
  data: torque input; torque output; rate input; dm parameter
function torque = torqueBox(torque,rate, dm)

momentum = dm.rw_mdl.moi * rate;
maxAngMom = dm.rw_mdl.maxAngMom;
AvlAngMom = dm.rw_mdl.avlAngMom;
maxTorque = dm.rw_mdl.maxTorque;

if momentum >= AvlAngMom && momentum <= maxAngMom
    torque = 1 + (-maxTorque) * (momentum);
elseif momentum <= -AvlAngMom && momentum >= (-maxAngMom)
    torque = -1 + (-maxTorque) * (momentum);
end

== matlab function B5G_SIM_PDR_ASH_V0/RWA/Nonlinear/RW4/MATLAB Function ==
  data: torque input; torque output; rate input; dm parameter
function torque = torqueBox(torque,rate, dm)

momentum = dm.rw_mdl.moi * rate;
maxAngMom = dm.rw_mdl.maxAngMom;
AvlAngMom = dm.rw_mdl.avlAngMom;
maxTorque = dm.rw_mdl.maxTorque;

if momentum >= AvlAngMom && momentum <= maxAngMom
    torque = 1 + (-maxTorque) * (momentum);
elseif momentum <= -AvlAngMom && momentum >= (-maxAngMom)
    torque = -1 + (-maxTorque) * (momentum);
end

== matlab function B5G_SIM_PDR_ASH_V0/Space Environment Models/MagneticField/Variant Subsystem/MagneticDipoleModel ==
  data: Pecf input; BnT output; dm parameter
function BnT = MagDipole(Pecf, dm)

BnT = MagneticDipole(Pecf, dm.mpm);

== matlab function B5G_SIM_PDR_ASH_V0/Spacecraft/Disturbance Models/Aerodynamics ==
  data: t_aero_total output; f_aero output; V input; dm parameter
function [t_aero_total, f_aero] = Aerodynamics(V,dm)
    f_aero = zeros(length(dm.norV),3);
    t_aero = zeros(length(dm.norV),3);
    for i = 1:length(dm.norV)
        if dot(dm.norV(i,:),V)>0
        f_aero(i,:) = -0.5 * dm.aeroCoeffDrag * dm.airDensity * norm(V)^2 * dm.area(i)*1e-6 * dot(dm.norV(i,:),V/norm(V)) *V/norm(V);
        t_aero(i,:) = cross(dm.rs(i,:),f_aero(i,:));
        end    
    end
     t_aero_total = sum(t_aero)';
end

== matlab function B5G_SIM_PDR_ASH_V0/Spacecraft/Disturbance Models/Gravity-Gradient Torque ==
  data: Rs input; tao_grav output; dm parameter
function tao_grav = dist_gravity(Rs, dm)

% from Wertx p567
% Rs_hat = ECI Position unit vector in body frame
Rs_hat = -Rs/norm(Rs);
tao_grav = ((3*dm.mu_e/norm(Rs)^3)*cross(Rs_hat, dm.Ib*Rs_hat));

== matlab function B5G_SIM_PDR_ASH_V0/Spacecraft/Disturbance Models/Solar pressure ==
  data: t_solar_total output; f_solar output; S input; dm parameter; Eclipse input
function [t_solar_total,f_solar ] = SolarPressure(S,dm, Eclipse)
    f_solar = zeros(length(dm.norV),3);
    t_solar = zeros(length(dm.norV),3);
    if Eclipse ==0
        for i = 1:length(dm.norV)
            if dot(dm.norV(i,:),S)>0
            f_solar(i,:) = -dm.P*dm.area(i)*1e-6*dot(dm.norV(i,:),S)*...
                ((1-dm.Cs)*S' + 2*(dm.Cd/3 + dm.Cs*dot(dm.norV(i,:),S))*dm.norV(i,:));
            t_solar(i,:) = cross(dm.rs(i,:),f_solar(i,:));
            end
        end
    end
    t_solar_total = sum(t_solar)';
end

== matlab function B5G_SIM_PDR_ASH_V0/Spacecraft/Disturbance Models/Subsystem/ECI to Body ==
  data: Va input; Qa2b input; Vb output
function Vb = EciToBody(Va,Qa2b)
Qb2a = QInv(Qa2b);
qout = QMul(QMul(Qb2a, [0;Va]), Qa2b);
Vb   = [qout(2) qout(3) qout(4)]';

== matlab function B5G_SIM_PDR_ASH_V0/RW_CTRL_FUN/Angular momentum Estimate ==
  settings: updateMethod=DISCRETE
  data: w_rpm input; tc input; h output; fsw parameter
function h = fcn(w_rpm,tc, fsw) %[C0, h]
persistent hrw

if isempty(hrw)
    hrw = fsw.rw.eqpt.H0;
end

rpm2rads    = (2*pi)/60;
J           = fsw.rw.eqpt.MOI; %parm(1); % 0.00663; %kg-m2 from 2ICD2885 Rev C August 2019
Te          = fsw.dt; %parm(2); % control period
w_est       = 0.52/10;

w = w_rpm*rpm2rads; 
h = hrw + 1.4 * w_est *Te*(J.*w-hrw);
hrw = h + Te*tc;
% h = J*w-h0;

== matlab function B5G_SIM_PDR_ASH_V0/Spacecraft/Disturbance Models/Subsystem/SunEci to SunSc ==
  data: Va input; Qa2b input; Vb output
function Vb = EciToBody(Va,Qa2b)
Qb2a = QInv(Qa2b);
qout = QMul(QMul(Qb2a, [0;Va]), Qa2b);
Vb   = [qout(2) qout(3) qout(4)]';
